simulink model "BB8"  (R2015b)
settings: Solver=VariableStepAuto  StartTime=0.0  StopTime=30  RelTol=1e-3
libraries: simulink x3
settings Model: Creator=msearing  LastModifiedBy=zoefiddler

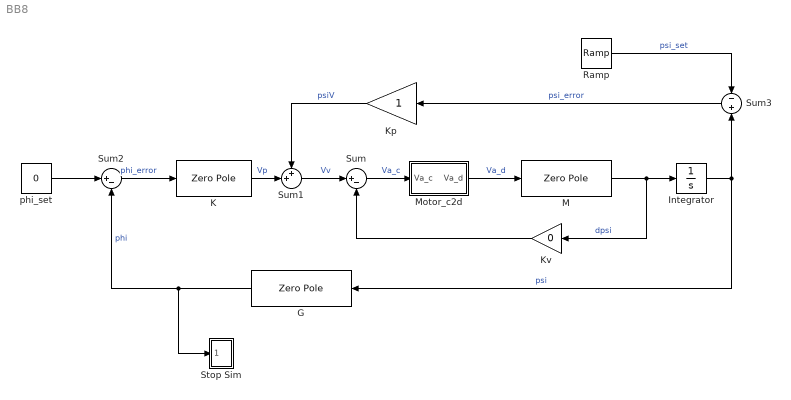
== system BB8 ==
  G : ZeroPole  Zeros="[0           0]"  Poles="[1.7694     -1.7694]"  Gain=[-0.026326]
  Integrator : Integrator
  K : ZeroPole  Zeros=[-1.5]  Poles=[-0.1]  Gain=[-333.33]
  Kp : Gain
  Kv : Gain  Gain=0
  M : ZeroPole  Zeros=[]  Poles=[-427.53]  Gain=[700.85]
  Motor_c2d : Subsystem
  Ramp : simulink/Sources/Ramp  slope=10  start=1  X0=0
  Stop Sim : Subsystem
  Sum : Sum  Inputs=|+-
  Sum1 : Sum  Inputs=++|
  Sum2 : Sum  Inputs=|+-
  Sum3 : Sum  Inputs=-|+
  phi_set : Constant  Value=0
  wires:
  M/1 -> Integrator/1, Kv/1  "dpsi"
  Kv/1 -> Sum/2
  Integrator/1 -> G/1, Sum3/2  "psi"
  Sum1/1 -> Sum/1  "Vv"
  K/1 -> Sum1/2  "Vp"
  G/1 -> Stop Sim/1(Phi), Sum2/2  "phi"
  Sum2/1 -> K/1  "phi_error"
  phi_set/1 -> Sum2/1
  Sum3/1 -> Kp/1  "psi_error"
  Kp/1 -> Sum1/1  "psiV"
  Ramp/1 -> Sum3/1  "psi_set"
  Sum/1 -> Motor_c2d/1(Va_c)  "Va_c"
  Motor_c2d/1(Va_d) -> M/1  "Va_d"

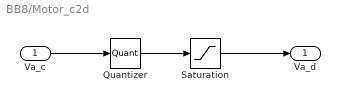
== system BB8/Motor_c2d ==
  Va_c : Inport
  Quantizer : Quantizer  QuantizationInterval=12/255
  Saturation : Saturate  UpperLimit=12  LowerLimit=-12
  Va_d : Outport
  wires:
  Saturation/1 -> Va_d/1
  Va_c/1 -> Quantizer/1
  Quantizer/1 -> Saturation/1

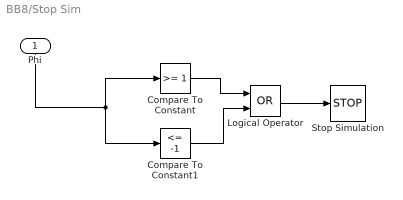
== system BB8/Stop Sim ==
  Phi : Inport
  Compare To Constant : simulink/Logic and Bit Operations/Compare To Constant  relop=>=  const=1  OutDataTypeStr=boolean
  Compare To Constant1 : simulink/Logic and Bit Operations/Compare To Constant  relop=<=  const=-1  OutDataTypeStr=boolean
  Logical Operator : Logic  Operator=OR  AllPortsSameDT=off  OutDataTypeStr=boolean
  Stop Simulation : Stop
  wires:
  Compare To Constant1/1 -> Logical Operator/2
  Logical Operator/1 -> Stop Simulation/1
  Compare To Constant/1 -> Logical Operator/1
  Phi/1 -> Compare To Constant/1, Compare To Constant1/1
